simulink model "PendulumSimulation"  (R2016b)
settings: Solver=ode45  StartTime=0.0  StopTime=tF  RelTol=1e-3  EnableMultiTasking=on
undefined symbols (not defined in the file): friction, g, l, x0
settings Model: Creator=pedropereira  LastModifiedBy=pedropereira
settings DataIOCC: LimitDataPoints=on  SaveFormat=Array
settings OptimizationCC: LifeSpan=inf
settings DebuggingCC: SolverPrmCheckMsg=warning  SFUnexpectedBacktrackingDiag=warning  SFNoUnconditionalDefaultTransitionDiag=warning  SFExecutionAtInitializationDiag=none
settings HardwareCC: ProdBitPerPointer=32  ProdBitPerSizeT=32  ProdBitPerPtrDiffT=32  ProdLargestAtomicFloat=None  ProdIntDivRoundTo=Undefined  ProdEndianess=Unspecified  ProdWordSize=32  ProdHWDeviceType=32-bit Generic
settings ModelReferenceCC: PropagateSignalLabelsOutOfModel=off
settings GRTTargetCC: TargetLangStandard=C89/C90 (ANSI)  GeneratePreprocessorConditionals=Disable all
settings ConfigComp: CovMetricSettings=dw  CovHtmlReporting=on  CovSaveCumulativeToWorkspaceVar=on  CovSaveSingleToWorkspaceVar=on  CovExternalEMLEnable=off  CovSFcnEnable=off

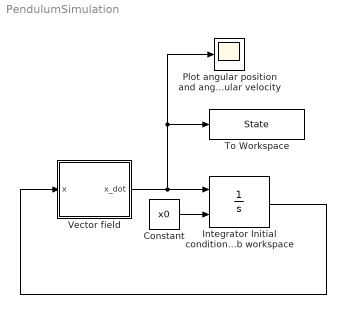
== system PendulumSimulation ==
  Constant : Constant  Value=x0
  Integrator Initial condition comes from matlab workspace : Integrator  InitialConditionSource=external
  Plot angular position and angular velocity : Scope
  To Workspace : ToWorkspace  VariableName=State  SaveFormat=Timeseries  SampleTime=-1
  Vector field : MATLAB Function  TreatAsAtomicUnit=on
  wires:
  Integrator Initial condition comes from matlab workspace/1 -> Vector field/1(x)
  Constant/1 -> Integrator Initial condition comes from matlab workspace/2
  Vector field/1(x_dot) -> To Workspace/1, Plot angular position and angular velocity/1, Integrator Initial condition comes from matlab workspace/1

== matlab function PendulumSimulation/Vector field ==
  data: x input; g parameter; l parameter; x_dot output; friction parameter
function x_dot = vector_field(x,g,l,friction)
% in EDITOR TAB->Edit Data, alter SCOPE from Input to Parameter
% this way g,l and k come from matlab workspace
% only real input is state x

% Repeat vector field here
x_dot = [x(2); -g/l*sin(x(1)) - friction*l*x(2)];
